simulink model "HAE"  (R2018a)
settings: Solver=ode4  StartTime=0  StopTime=2  MaxStep=1e-4  RelTol=1e-3
InitFcn:
  | close
  | clear
  | clc
  | Sc=128
  | f=60;
  | T=1/f;
  | Ts=1/(f*Sc);
  | Vr=6500
  | V_v=[1    0.4    1          0.6       1       0.6       1       0.75   0.95]
  | T_v=[0   20/f  70/f    200/f   300/f     330/f   400/f   500/f  10]
  | S_time=60/f*20.5
  | V_R=3;
  | Tf=3
  | T_lc=3
  | set_param('HAE/EMISOR-RECEPTOR/TCP_IP_RX1/ESCRITURA', 'Value','0')
  | set_param('HAE/EMISOR-RECEPTOR/TCP_IP_RX1/RETARDO', 'Value','0')
  | run script_client_1_inicio2.m
undefined symbols (not defined in the file or in its folder): D11, Delta, DiscIntNeverNeededParam, Int, Ip1
libraries: powerlib x68, simulink x12, powerlib_meascontrol x6, libreria_comunicaciones_cliente2 x2, libreria_medidores2 x1
(part 5 of 5)

== system HAE/Subsystem9/RMS ==
  In1 : Inport
  Absolute : MATLABFcn  MATLABFcn=abs
  Check zero Crossing : HitCross
  Constant : Constant  Value=F
  Derivative : Derivative
  Divide : Product  Inputs=/*
  Gain : Gain  Gain=2*pi
  Gain1 : Gain  Gain=1/sqrt(2)
  Hold derivative till next zero crossing : Subsystem  AncestorBlock=|  DialogController=POWERSYS.PowerSysDialog  mask(Discrete Sample & Hold){ic=0, Ts=-1}
      | powerlib_extras/Discrete 
      | Control Blocks/Discrete
      | Sample & Hold
      mask prompts: ic "Initial condition:"; Ts "Sample time:"
      mask help: The output follows input 1 (In) as long as input 2 (S) is TRUE (1) . The output is held when input 2 becomes FALSE (0). The output initial value is specified by the parameter "Initial condition".
      mask init:
      | power_initmask();
      mask Help: This block is part of a subset of blocks in the Extras library that does not have documentation associated with it, other than the block mask description.
      mask Display: disp('S/H')
  Out1 : Outport
  wires:
  Derivative/1 -> Hold derivative till next zero crossing/1(In)
  Check zero Crossing/1 -> Hold derivative till next zero crossing/2(S)
  Hold derivative till next zero crossing/1("   ") -> Absolute/1
  Constant/1 -> Gain/1
  Gain/1 -> Divide/1
  Absolute/1 -> Divide/2
  In1/1 -> Check zero Crossing/1, Derivative/1
  Divide/1 -> Gain1/1
  Gain1/1 -> Out1/1

== system HAE/Subsystem9/Timer Proteccion ==
  Entrada : Inport
  Pick-Up : Inport  Port=2
  T.O. : Inport  Port=3
  Arranq3 : Switch  Criteria=u2 ~= 0  Threshold=Ip1
  Arranq6 : Switch  Criteria=u2 ~= 0  Threshold=Ip1  ZeroCross=off
  C14 : Constant  Value=0
  C15 : Constant  Value=1000
  C16 : Constant
  Condicion arranque1 : RelationalOperator  Operator=>  OutDataTypeStr=boolean  RndMeth=Nearest
  Discrete-Time Integrator : DiscreteIntegrator  ExternalReset=falling  SampleTime=-1  ICPrevOutput=DiscIntNeverNeededParam  ICPrevScaledInput=DiscIntNeverNeededParam
  Logical Operator4 : Logic  Operator=NOT  AllPortsSameDT=off  OutDataTypeStr=boolean
  Tiempo Disparo1 : RelationalOperator  Operator=>  OutDataTypeStr=boolean  RndMeth=Nearest
  Trip : Outport
  wires:
  C16/1 -> Arranq6/1
  Arranq6/1 -> Logical Operator4/1, Arranq6/3
  Tiempo Disparo1/1 -> Arranq6/2
  T.O./1 -> Tiempo Disparo1/2
  C15/1 -> Arranq3/1
  C14/1 -> Arranq3/3
  Arranq3/1 -> Discrete-Time Integrator/1
  Condicion arranque1/1 -> Arranq3/2, Discrete-Time Integrator/2
  Pick-Up/1 -> Condicion arranque1/2
  Entrada/1 -> Condicion arranque1/1
  Discrete-Time Integrator/1 -> Tiempo Disparo1/1
  Logical Operator4/1 -> Trip/1

== system HAE/Subsystem9/Timer Proteccion1 ==
  Entrada : Inport
  Pick-Up : Inport  Port=2
  T.O. : Inport  Port=3
  Arranq3 : Switch  Criteria=u2 ~= 0  Threshold=Ip1
  Arranq6 : Switch  Criteria=u2 ~= 0  Threshold=Ip1  ZeroCross=off
  C14 : Constant  Value=0
  C15 : Constant  Value=1000
  C16 : Constant
  Condicion arranque1 : RelationalOperator  Operator=>  OutDataTypeStr=boolean  RndMeth=Nearest
  Discrete-Time Integrator : DiscreteIntegrator  ExternalReset=falling  SampleTime=-1  ICPrevOutput=DiscIntNeverNeededParam  ICPrevScaledInput=DiscIntNeverNeededParam
  Logical Operator4 : Logic  Operator=NOT  AllPortsSameDT=off  OutDataTypeStr=boolean
  Scope1 : Scope  NumInputPorts=2
  Tiempo Disparo1 : RelationalOperator  Operator=>  OutDataTypeStr=boolean  RndMeth=Nearest
  Trip : Outport
  wires:
  C16/1 -> Arranq6/1
  Arranq6/1 -> Logical Operator4/1, Arranq6/3
  Tiempo Disparo1/1 -> Arranq6/2
  T.O./1 -> Tiempo Disparo1/2
  C15/1 -> Arranq3/1
  C14/1 -> Arranq3/3
  Arranq3/1 -> Discrete-Time Integrator/1
  Condicion arranque1/1 -> Scope1/1, Arranq3/2, Discrete-Time Integrator/2
  Pick-Up/1 -> Condicion arranque1/2
  Entrada/1 -> Condicion arranque1/1
  Discrete-Time Integrator/1 -> Scope1/2, Tiempo Disparo1/1
  Logical Operator4/1 -> Trip/1

== system HAE/Articulo 2 1/Hyperbolic model/counter1 ==
  In2 : Inport
  Add3 : Sum
  Arranq1 : Switch  Threshold=2  ZeroCross=off
  Constant1 : Constant  Value=Ts
  Constant2 : Constant
  Constant5 : Constant  Value=0
  Divide : Product  Inputs=**
  Unit Delay1 : UnitDelay  SampleTime=-1
  Unit Delay2 : UnitDelay  SampleTime=-1
  Counter Melting : Outport
  wires:
  Arranq1/1 -> Divide/2
  In2/1 -> Arranq1/2
  Constant5/1 -> Arranq1/3
  Constant2/1 -> Arranq1/1
  Add3/1 -> Counter Melting/1, Divide/1
  Divide/1 -> Unit Delay1/1
  Unit Delay1/1 -> Add3/2
  Unit Delay2/1 -> Add3/1
  Constant1/1 -> Unit Delay2/1

== system HAE/Articulo 2 1/Hyperbolic model/counter2 ==
  Add3 : Sum
  Arranq3 : Switch  Threshold=1.5  ZeroCross=off
  Constant1 : Constant  Value=Ts
  Constant3 : Constant  Value=0
  Constant4 : Constant
  Divide : Product  Inputs=**
  Unit Delay1 : UnitDelay  SampleTime=-1
  Unit Delay2 : UnitDelay  SampleTime=-1
  Counter Tap-to_Tap : Outport
  wires:
  Arranq3/1 -> Divide/2
  Add3/1 -> Counter Tap-to_Tap/1, Arranq3/2, Divide/1
  Divide/1 -> Unit Delay1/1
  Constant4/1 -> Arranq3/3
  Constant3/1 -> Arranq3/1
  Unit Delay1/1 -> Add3/2
  Unit Delay2/1 -> Add3/1
  Constant1/1 -> Unit Delay2/1

== system HAE/Articulo 2 1/Hyperbolic model1/counter1 ==
  In2 : Inport
  Add3 : Sum
  Arranq1 : Switch  Threshold=2  ZeroCross=off
  Constant1 : Constant  Value=Ts
  Constant2 : Constant
  Constant5 : Constant  Value=0
  Divide : Product  Inputs=**
  Unit Delay1 : UnitDelay  SampleTime=-1
  Unit Delay2 : UnitDelay  SampleTime=-1
  Counter Melting : Outport
  wires:
  Arranq1/1 -> Divide/2
  In2/1 -> Arranq1/2
  Constant5/1 -> Arranq1/3
  Constant2/1 -> Arranq1/1
  Add3/1 -> Counter Melting/1, Divide/1
  Divide/1 -> Unit Delay1/1
  Unit Delay1/1 -> Add3/2
  Unit Delay2/1 -> Add3/1
  Constant1/1 -> Unit Delay2/1

== system HAE/Articulo 2 1/Hyperbolic model1/counter2 ==
  Add3 : Sum
  Arranq3 : Switch  Threshold=1.5  ZeroCross=off
  Constant1 : Constant  Value=Ts
  Constant3 : Constant  Value=0
  Constant4 : Constant
  Divide : Product  Inputs=**
  Unit Delay1 : UnitDelay  SampleTime=-1
  Unit Delay2 : UnitDelay  SampleTime=-1
  Counter Tap-to_Tap : Outport
  wires:
  Arranq3/1 -> Divide/2
  Add3/1 -> Counter Tap-to_Tap/1, Arranq3/2, Divide/1
  Divide/1 -> Unit Delay1/1
  Constant4/1 -> Arranq3/3
  Constant3/1 -> Arranq3/1
  Unit Delay1/1 -> Add3/2
  Unit Delay2/1 -> Add3/1
  Constant1/1 -> Unit Delay2/1

== system HAE/Articulo 2 1/Hyperbolic model2/counter1 ==
  In2 : Inport
  Add3 : Sum
  Arranq1 : Switch  Threshold=2  ZeroCross=off
  Constant1 : Constant  Value=Ts
  Constant2 : Constant
  Constant5 : Constant  Value=0
  Divide : Product  Inputs=**
  Unit Delay1 : UnitDelay  SampleTime=-1
  Unit Delay2 : UnitDelay  SampleTime=-1
  Counter Melting : Outport
  wires:
  Arranq1/1 -> Divide/2
  In2/1 -> Arranq1/2
  Constant5/1 -> Arranq1/3
  Constant2/1 -> Arranq1/1
  Add3/1 -> Counter Melting/1, Divide/1
  Divide/1 -> Unit Delay1/1
  Unit Delay1/1 -> Add3/2
  Unit Delay2/1 -> Add3/1
  Constant1/1 -> Unit Delay2/1

== system HAE/Articulo 2 1/Hyperbolic model2/counter3 ==
  Add3 : Sum
  Arranq3 : Switch  Threshold=1.5  ZeroCross=off
  Constant1 : Constant  Value=Ts
  Constant3 : Constant  Value=0
  Constant4 : Constant
  Divide : Product  Inputs=**
  Unit Delay1 : UnitDelay  SampleTime=-1
  Unit Delay2 : UnitDelay  SampleTime=-1
  Counter Tap-to_Tap : Outport
  wires:
  Arranq3/1 -> Divide/2
  Add3/1 -> Counter Tap-to_Tap/1, Arranq3/2, Divide/1
  Divide/1 -> Unit Delay1/1
  Constant4/1 -> Arranq3/3
  Constant3/1 -> Arranq3/1
  Unit Delay1/1 -> Add3/2
  Unit Delay2/1 -> Add3/1
  Constant1/1 -> Unit Delay2/1

== system HAE/RB1/RMS1/Hold derivative till next zero crossing ==
  note: Silvano Casoria
      | Power System Simulation Laboratory
      | IREQ, Hydro-Quebc
  note: Sample and Hold
  In : Inport
  S : Inport  Port=2
  Memory : Memory
  Switch : Switch  Threshold=0.5  SaturateOnIntegerOverflow=on  InputSameDT=on
  "   " : Outport  InitialOutput=0
  wires:
  S/1 -> Switch/2
  In/1 -> Switch/1
  Memory/1 -> Switch/3
  Switch/1 -> Memory/1, "   "/1

== system HAE/RB1/RMS1/Hold derivative till next zero crossing1 ==
  note: Sample and Hold
  note: Silvano Casoria
      | Power System Simulation Laboratory
      | IREQ, Hydro-Quebc
  In : Inport
  S : Inport  Port=2
  Memory : Memory
  Switch : Switch  Threshold=0.5  SaturateOnIntegerOverflow=on  InputSameDT=on
  "   " : Outport  InitialOutput=0
  wires:
  Switch/1 -> "   "/1, Memory/1
  Memory/1 -> Switch/3
  In/1 -> Switch/1
  S/1 -> Switch/2

== system HAE/RB1/RMS1/Hold derivative till next zero crossing2 ==
  note: Silvano Casoria
      | Power System Simulation Laboratory
      | IREQ, Hydro-Quebc
  note: Sample and Hold
  In : Inport
  S : Inport  Port=2
  Memory : Memory
  Switch : Switch  Threshold=0.5  SaturateOnIntegerOverflow=on  InputSameDT=on
  "   " : Outport  InitialOutput=0
  wires:
  S/1 -> Switch/2
  In/1 -> Switch/1
  Memory/1 -> Switch/3
  Switch/1 -> Memory/1, "   "/1

== system HAE/RB4/RMS1/Hold derivative till next zero crossing ==
  note: Sample and Hold
  note: Silvano Casoria
      | Power System Simulation Laboratory
      | IREQ, Hydro-Quebc
  In : Inport
  S : Inport  Port=2
  Memory : Memory
  Switch : Switch  Threshold=0.5  SaturateOnIntegerOverflow=on  InputSameDT=on
  "   " : Outport  InitialOutput=0
  wires:
  Switch/1 -> "   "/1, Memory/1
  Memory/1 -> Switch/3
  In/1 -> Switch/1
  S/1 -> Switch/2

== system HAE/RB4/RMS1/Hold derivative till next zero crossing1 ==
  note: Silvano Casoria
      | Power System Simulation Laboratory
      | IREQ, Hydro-Quebc
  note: Sample and Hold
  In : Inport
  S : Inport  Port=2
  Memory : Memory
  Switch : Switch  Threshold=0.5  SaturateOnIntegerOverflow=on  InputSameDT=on
  "   " : Outport  InitialOutput=0
  wires:
  S/1 -> Switch/2
  In/1 -> Switch/1
  Memory/1 -> Switch/3
  Switch/1 -> Memory/1, "   "/1

== system HAE/RB4/RMS1/Hold derivative till next zero crossing2 ==
  note: Sample and Hold
  note: Silvano Casoria
      | Power System Simulation Laboratory
      | IREQ, Hydro-Quebc
  In : Inport
  S : Inport  Port=2
  Memory : Memory
  Switch : Switch  Threshold=0.5  SaturateOnIntegerOverflow=on  InputSameDT=on
  "   " : Outport  InitialOutput=0
  wires:
  Switch/1 -> "   "/1, Memory/1
  Memory/1 -> Switch/3
  In/1 -> Switch/1
  S/1 -> Switch/2

== system HAE/RB5/RMS1/Hold derivative till next zero crossing ==
  note: Silvano Casoria
      | Power System Simulation Laboratory
      | IREQ, Hydro-Quebc
  note: Sample and Hold
  In : Inport
  S : Inport  Port=2
  Memory : Memory
  Switch : Switch  Threshold=0.5  SaturateOnIntegerOverflow=on  InputSameDT=on
  "   " : Outport  InitialOutput=0
  wires:
  S/1 -> Switch/2
  In/1 -> Switch/1
  Memory/1 -> Switch/3
  Switch/1 -> Memory/1, "   "/1

== system HAE/RB5/RMS1/Hold derivative till next zero crossing1 ==
  note: Sample and Hold
  note: Silvano Casoria
      | Power System Simulation Laboratory
      | IREQ, Hydro-Quebc
  In : Inport
  S : Inport  Port=2
  Memory : Memory
  Switch : Switch  Threshold=0.5  SaturateOnIntegerOverflow=on  InputSameDT=on
  "   " : Outport  InitialOutput=0
  wires:
  Switch/1 -> "   "/1, Memory/1
  Memory/1 -> Switch/3
  In/1 -> Switch/1
  S/1 -> Switch/2

== system HAE/RB5/RMS1/Hold derivative till next zero crossing2 ==
  note: Silvano Casoria
      | Power System Simulation Laboratory
      | IREQ, Hydro-Quebc
  note: Sample and Hold
  In : Inport
  S : Inport  Port=2
  Memory : Memory
  Switch : Switch  Threshold=0.5  SaturateOnIntegerOverflow=on  InputSameDT=on
  "   " : Outport  InitialOutput=0
  wires:
  S/1 -> Switch/2
  In/1 -> Switch/1
  Memory/1 -> Switch/3
  Switch/1 -> Memory/1, "   "/1

== system HAE/Subsystem1/RMS/Hold derivative till next zero crossing ==
  note: Silvano Casoria
      | Power System Simulation Laboratory
      | IREQ, Hydro-Quebc
  note: Sample and Hold
  In : Inport
  S : Inport  Port=2
  Memory : Memory
  Switch : Switch  Threshold=0.5  SaturateOnIntegerOverflow=on  InputSameDT=on
  "   " : Outport  InitialOutput=0
  wires:
  S/1 -> Switch/2
  In/1 -> Switch/1
  Memory/1 -> Switch/3
  Switch/1 -> Memory/1, "   "/1

== system HAE/Subsystem10/RMS/Hold derivative till next zero crossing ==
  note: Silvano Casoria
      | Power System Simulation Laboratory
      | IREQ, Hydro-Quebc
  note: Sample and Hold
  In : Inport
  S : Inport  Port=2
  Memory : Memory
  Switch : Switch  Threshold=0.5  SaturateOnIntegerOverflow=on  InputSameDT=on
  "   " : Outport  InitialOutput=0
  wires:
  S/1 -> Switch/2
  In/1 -> Switch/1
  Memory/1 -> Switch/3
  Switch/1 -> Memory/1, "   "/1

== system HAE/Subsystem3/RMS/Hold derivative till next zero crossing ==
  note: Silvano Casoria
      | Power System Simulation Laboratory
      | IREQ, Hydro-Quebc
  note: Sample and Hold
  In : Inport
  S : Inport  Port=2
  Memory : Memory
  Switch : Switch  Threshold=0.5  SaturateOnIntegerOverflow=on  InputSameDT=on
  "   " : Outport  InitialOutput=0
  wires:
  S/1 -> Switch/2
  In/1 -> Switch/1
  Memory/1 -> Switch/3
  Switch/1 -> Memory/1, "   "/1

== system HAE/Subsystem6/RMS/Hold derivative till next zero crossing ==
  note: Silvano Casoria
      | Power System Simulation Laboratory
      | IREQ, Hydro-Quebc
  note: Sample and Hold
  In : Inport
  S : Inport  Port=2
  Memory : Memory
  Switch : Switch  Threshold=0.5  SaturateOnIntegerOverflow=on  InputSameDT=on
  "   " : Outport  InitialOutput=0
  wires:
  S/1 -> Switch/2
  In/1 -> Switch/1
  Memory/1 -> Switch/3
  Switch/1 -> Memory/1, "   "/1

== system HAE/Subsystem7/RMS/Hold derivative till next zero crossing ==
  note: Silvano Casoria
      | Power System Simulation Laboratory
      | IREQ, Hydro-Quebc
  note: Sample and Hold
  In : Inport
  S : Inport  Port=2
  Memory : Memory
  Switch : Switch  Threshold=0.5  SaturateOnIntegerOverflow=on  InputSameDT=on
  "   " : Outport  InitialOutput=0
  wires:
  S/1 -> Switch/2
  In/1 -> Switch/1
  Memory/1 -> Switch/3
  Switch/1 -> Memory/1, "   "/1

== system HAE/Subsystem8/RMS/Hold derivative till next zero crossing ==
  note: Silvano Casoria
      | Power System Simulation Laboratory
      | IREQ, Hydro-Quebc
  note: Sample and Hold
  In : Inport
  S : Inport  Port=2
  Memory : Memory
  Switch : Switch  Threshold=0.5  SaturateOnIntegerOverflow=on  InputSameDT=on
  "   " : Outport  InitialOutput=0
  wires:
  S/1 -> Switch/2
  In/1 -> Switch/1
  Memory/1 -> Switch/3
  Switch/1 -> Memory/1, "   "/1

== system HAE/Subsystem9/RMS/Hold derivative till next zero crossing ==
  note: Silvano Casoria
      | Power System Simulation Laboratory
      | IREQ, Hydro-Quebc
  note: Sample and Hold
  In : Inport
  S : Inport  Port=2
  Memory : Memory
  Switch : Switch  Threshold=0.5  SaturateOnIntegerOverflow=on  InputSameDT=on
  "   " : Outport  InitialOutput=0
  wires:
  S/1 -> Switch/2
  In/1 -> Switch/1
  Memory/1 -> Switch/3
  Switch/1 -> Memory/1, "   "/1
